simulink library "DQ_SR_LIB_SIM"  (R2015b)
settings: Solver=VariableStepAuto  StartTime=0.0  StopTime=10.0  RelTol=1e-3
undefined symbols (not defined in the file or in its folder): crossqm, II, magnitude, X0, XCG0, xi0
undefined symbols (not defined in the file): II0, SATFUNCNAME
(part 2 of 2)

== matlab function DQ_SR_LIB_SIM/Utilities/quaternion product/MATLAB Function ==
  data: u input; y output; fun_NAME parameter; ISTRANSPOSE parameter
function y = fcn(u,fun_NAME,ISTRANSPOSE)
%#codegen

% extract function
fun=str2func(char(fun_NAME));
% evaluate function
y = fun(u);

if ISTRANSPOSE
   % traspose if required 
    y = y';
end

== matlab function DQ_SR_LIB_SIM/Utilities/dual quaternion product/MATLAB Function ==
  data: u input; y output; fun_NAME parameter; ISTRANSPOSE parameter
function y = fcn(u,fun_NAME,ISTRANSPOSE)
%#codegen

% extract function
fun=str2func(char(fun_NAME));
% evaluate function
y = fun(u);

if ISTRANSPOSE
   % traspose if required 
    y = y';
end

== matlab function DQ_SR_LIB_SIM/Utilities/Inertial dq/MATLAB Function ==
  data: a output; d input; q input
function a = fcn(d,q)
%#codegen


QM=crossqm(q);
QM=QM(:,1:3);

t = QM*d/2;

a = [q;t];

== matlab function DQ_SR_LIB_SIM/Utilities/dq normalizer/MATLAB Function ==
  data: u input; y output
function y = fcn(u)
%#codegen

% input
q = u(1:4);
t = u(5:8);

% normalize attitude quaternion
q = q/norm(q);

% normalize position quaternion
d = 2*crossqm(q)'*t;
t = .5*crossqm(q)*[d(1:3);0];

%output
y = [q;t];

== matlab function DQ_SR_LIB_SIM/Utilities/Dual quaternion selection/MATLAB Function ==
  data: a input; x parameter; y parameter; a_xy output
function a_xy = selectindex(a,x,y)
%#codegen
% select as output the index of elements and body

[~,n]=size(a);

if n==1
    % avoid null selection
    y=1;
end

% a_xy=zeros(8,8);

a_xy = a(x,y);
